simulink model "norton_5_nl_push_pull"  (Simulink 7.4)
settings: Solver=ode23t  StartTime=0.0  StopTime=1e-4  MaxStep=10e-9  RelTol=1e-4
InitFcn:
  | M=3;
  | N=M^2-M-1;
  | 
  | L1=1e-6;
  | R1=0.1;
  | L2=(M^2)*L1;
  | R2=R1*M;
  | L3=(N^2)*L1;
  | R3=R1*N;
  | 
  | K=0.999;
  | M12 = K*sqrt(L1*L2);
  | M13 = K*sqrt(L1*L3);
  | M23 = K*sqrt(L2*L3);
  | 
  | % center tapped input transformer
  | Kio = 0.999;
  | Lio1 = 4e-6;
  | Lio2   = Lio1*(0.5^2);
  | Lio3   = Lio2;
  | Mio12 = Kio*sqrt(Lio1*Lio2);
  | Mio13 = Kio*sqrt(Lio1*Lio3);
  | Mio23 = Kio*sqrt(Lio2*Lio3);
  | Rio = 1;
  | 
  | % Passive Augmentation Transformer
  | La1 = 1e-6;
  | Ka=0.9999;
  | Tratio = 5;
  | La2 = La1*(Tratio^2);
  | Ma12 = Ka*Tratio*La1;
  | Ra1=0.1;
  | Ra2=Tratio*Ra1;
StopFcn:
  | if ~SPECTRUM_FLAG
  |      %% plot measured sparameters using RFTB
  |     amp=rfdata.data;
  |     amp.Freq=spar(:,1);
  | %%
  |     amp.S_parameters=complex(zeros(2,2,length(amp.Freq)));
  |    if spar(1,6)==1
  |       amp.S_Parameters(1,1,:)=spar(:,2)+1i*spar(:,3);
  |       amp.S_Parameters(2,1,:)=spar(:,4)+1i*spar(:,5);
  |       subplot(2,1,1);
  |       hplot1= smith(amp,'s11')
  |       subplot(2,1,2);
  |       hplot2 = plot(amp,'s21');
  |       axis([amp.Freq(1)/1e6,amp.Freq(end)/1e6,0,10]);
  |    else
  |       amp.S_Parameters(2,2,:)=spar(:,2)+1i*spar(:,3);
  |       amp.S_Parameters(1,2,:)=spar(:,4)+1i*spar(:,5);
  |       subplot(2,1,1);
  |       hplot1= smith(amp,'s22')
  |       subplot(2,1,2);
  |       hplot2 = plot(amp,'s12');
  |    end;
  | end
undefined symbols (not defined in the file or in its folder): Fs, magnitude, One, sided
libraries: powerlib x65, dspindex x12, dspsigops x6, dspbuff3 x5, dsparch4 x5, simulink x4, dspxfrm3 x4, dsparch3 x4, dspsnks4 x3, dspmtrx3 x2, dspstat3 x1
(part 1 of 2)
settings Model: Creator=Dick  LastModifiedBy=Dick

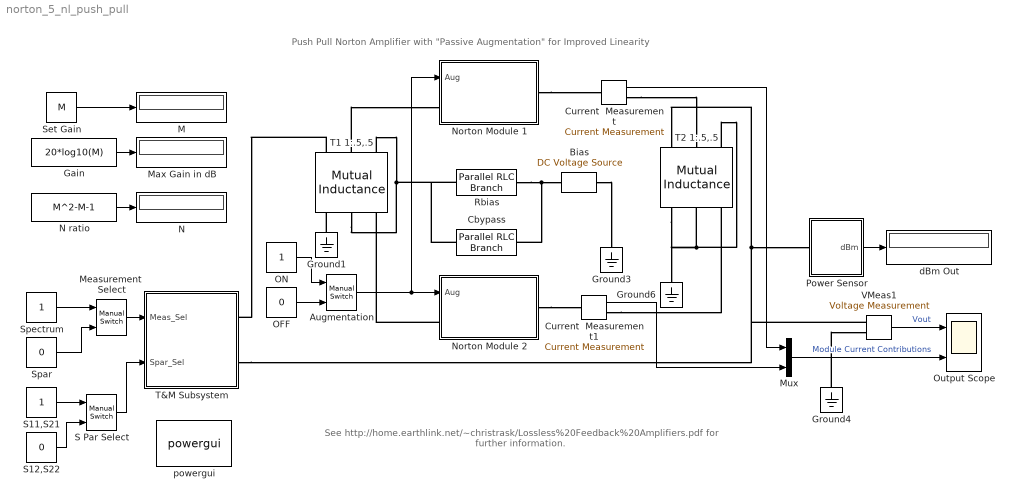
== system norton_5_nl_push_pull ==
  note: Push Pull Norton Amplifier with "Passive Augmentation" for Improved Linearity
  note: See http://home.earthlink.net/~christrask/Lossless%20Feedback%20Amplifiers.pdf
      | for further information.
  Augmentation : simulink/Signal Routing/Manual Switch  SystemSampleTime=-1  sw=0  action=0  varsize=off
  Bias : powerlib/Electrical Sources/DC Voltage Source  DialogController=POWERSYS.PowerSysDialog  SystemSampleTime=-1  Amplitude=3  Measurements=None
  Cbypass : powerlib/Elements/Parallel RLC Branch  DialogController=POWERSYS.PowerSysDialog  PhysicalDomain=powersysdomain  SubClassName=unknown  LeftPortType=p1  RightPortType=p1  LConnTagsString=a  RConnTagsString=__new0  BranchType=C  Resistance=.01  Inductance=1e-3  SetiL0=off  InitialCurrent=0  Capacitance=1e-7  Setx0=off  InitialVoltage=0  Measurements=None
  Current  Measurement : powerlib/Measurements/Current Measurement  DialogController=POWERSYS.PowerSysDialog  SystemSampleTime=-1  PhasorSimulation=off  OutputType=Complex  PSBequivalent=0
  Current  Measurement1 : powerlib/Measurements/Current Measurement  DialogController=POWERSYS.PowerSysDialog  SystemSampleTime=-1  PhasorSimulation=off  OutputType=Complex  PSBequivalent=0
  Gain : Constant  Value=20*log10(M)  OutDataType=fixdt(1, 16)  OutScaling=2^0
  Ground{1,3..4,6} (4 alike) : powerlib/Elements/Ground  DialogController=POWERSYS.PowerSysDialog  PhysicalDomain=powersysdomain  SubClassName=unknown  LeftPortType=p1  RightPortType=p1  LConnTagsString=a
  M : Display
  Max Gain in dB : Display
  Measurement  Select : simulink/Signal Routing/Manual Switch  SystemSampleTime=-1  sw=1  action=0  varsize=off
  Mux : Mux  Inputs=2
  N : Display
  N ratio : Constant  Value=M^2-M-1  OutDataType=fixdt(1, 16)  OutScaling=2^0
  Norton Module 1 : Subsystem
  Norton Module 2 : Subsystem
  OFF : Constant  Value=0  OutDataType=fixdt(1, 16)  OutScaling=2^0
  ON : Constant  OutDataType=fixdt(1, 16)  OutScaling=2^0
  Output Scope : Scope  NumInputPorts=2
      settings: TimeRange=5.999999999999993e-007  YMin=-30~-0.3  YMax=30~1.2
  Power Sensor : Subsystem
  Rbias : powerlib/Elements/Parallel RLC Branch  DialogController=POWERSYS.PowerSysDialog  PhysicalDomain=powersysdomain  SubClassName=unknown  LeftPortType=p1  RightPortType=p1  LConnTagsString=a  RConnTagsString=__new0  BranchType=R  Resistance=50/2  Inductance=1e-3  SetiL0=off  InitialCurrent=0  Capacitance=1e-6  Setx0=off  InitialVoltage=0  Measurements=None
  S Par Select : simulink/Signal Routing/Manual Switch  SystemSampleTime=-1  sw=1  action=0  varsize=off
  S11,S21 : Constant  OutDataType=fixdt(1, 16)  OutScaling=2^0
  S12,S22 : Constant  Value=0  OutDataType=fixdt(1, 16)  OutScaling=2^0
  Set Gain : Constant  Value=M  OutDataType=fixdt(1, 16)  OutScaling=2^0
  Spar : Constant  Value=0  OutDataTypeMode=boolean  OutDataType=fixdt(1, 16)  OutScaling=2^0  OutDataTypeStr=boolean
  Spectrum : Constant  OutDataTypeMode=boolean  OutDataType=fixdt(1, 16)  OutScaling=2^0  OutDataTypeStr=boolean
  T&M Subsystem : Subsystem
  T1 1:.5,.5 : powerlib/Elements/Mutual Inductance  DialogController=POWERSYS.PowerSysDialog  PhysicalDomain=powersysdomain  SubClassName=unknown  LeftPortType=p1  RightPortType=p1  LConnTagsString=a|b|c  RConnTagsString=A|B|C  TypeOfMutual=Generalized mutual inductance  NumberOfWindings=3  SelfImpedance1=[R1,L1]  SelfImpedance2=[R2,L2]  ThreeWindings=on  SelfImpedance3=[]  MutualImpedance=[1.0 1.0e-03]  InductanceMatrix=[Lio1 Mio12 Mio13; Mio12 Lio2 Mio23; Mio13 Mio23 Lio3];  ResistanceMatrix="[1  0 0 ; 0 1 0 ; 0 0 1]*Rio;"  Measurements=None
      settings: AttributesFormatString=\n
  T2 1:.5,.5 : powerlib/Elements/Mutual Inductance  DialogController=POWERSYS.PowerSysDialog  PhysicalDomain=powersysdomain  SubClassName=unknown  LeftPortType=p1  RightPortType=p1  LConnTagsString=a|b|c  RConnTagsString=A|B|C  TypeOfMutual=Generalized mutual inductance  NumberOfWindings=3  SelfImpedance1=[R1,L1]  SelfImpedance2=[R2,L2]  ThreeWindings=on  SelfImpedance3=[]  MutualImpedance=[1.0 1.0e-03]  InductanceMatrix=[Lio1 Mio12 Mio13; Mio12 Lio2 Mio23; Mio13 Mio23 Lio3];  ResistanceMatrix="[1  0 0 ; 0 1 0 ; 0 0 1]*Rio;"  Measurements=None
      settings: AttributesFormatString=\n
  VMeas1 : powerlib/Measurements/Voltage Measurement  DialogController=POWERSYS.PowerSysDialog  SystemSampleTime=-1  PhasorSimulation=off  OutputType=Complex  PSBequivalent=0
  dBm Out : Display
  powergui : powerlib/powergui  Priority=1  SystemSampleTime=-1  SimulationMode=Continuous  SampleTime=50e-6  frequency=60  SPID=off  DisableSnubberDevices=off  DisableRonSwitches=off  DisableVfSwitches=off  SwTol=0  Interpol=off  frequencyindice=0  echomessages=off  HookPort=off  DisplayEquations=off  FunctionMessages=off  EnableUseOfTLC=off  x0status=blocks  RestoreLinks=warning  Frange=[0:2:500]  Ylog=off  Xlog=on  ShowGrid=off  save=off  variable=ZData  ZoomFFT=on  StartTime=0.0  cycles=1  DisplayStyle=1  fundamental=60  FreqAxis=off  MaxFrequency=1000  frequencyindicesteady=1  RmsSteady=1  display=off  Ts=0  methode=off
  wires:
  Set Gain/1 -> M/1
  N ratio/1 -> N/1
  Gain/1 -> Max Gain in dB/1
  ON/1 -> Augmentation/1
  OFF/1 -> Augmentation/2
  Augmentation/1 -> Norton Module 1/1(Aug), Norton Module 2/1(Aug)
  Measurement  Select/1 -> T&M Subsystem/1(Meas_Sel)
  Spar/1 -> Measurement  Select/2
  Spectrum/1 -> Measurement  Select/1
  S Par Select/1 -> T&M Subsystem/2(Spar_Sel)
  S11,S21/1 -> S Par Select/1
  S12,S22/1 -> S Par Select/2
  Current  Measurement/1 -> Mux/1
  Current  Measurement1/1 -> Mux/2
  Mux/1 -> Output Scope/2  "Module Current Contributions"
  VMeas1/1 -> Output Scope/1  "Vout"
  Power Sensor/1(dBm) -> dBm Out/1
  connections:
  Ground1/LConn1 -- T1 1:.5,.5/RConn1
  T1 1:.5,.5/LConn2 -- Norton Module 1/LConn1
  Bias/LConn1 -- Ground3/LConn1
  Norton Module 2/LConn1 -- T1 1:.5,.5/RConn3
  T1 1:.5,.5/LConn3 -- T1 1:.5,.5/RConn2 -- Rbias/LConn1 -- Cbypass/RConn1
  Rbias/RConn1 -- Bias/RConn1 -- Cbypass/LConn1
  T2 1:.5,.5/RConn1 -- Ground6/LConn1 -- T2 1:.5,.5/RConn2 -- T2 1:.5,.5/LConn3
  T1 1:.5,.5/LConn1 -- T&M Subsystem/RConn1
  T&M Subsystem/RConn2 -- VMeas1/LConn1 -- T2 1:.5,.5/LConn1 -- Power Sensor/LConn1
  Norton Module 1/RConn1 -- Current  Measurement/LConn1
  Current  Measurement/RConn1 -- T2 1:.5,.5/LConn2
  Norton Module 2/RConn1 -- Current  Measurement1/LConn1
  Current  Measurement1/RConn1 -- T2 1:.5,.5/RConn3
  Ground4/LConn1 -- VMeas1/LConn2

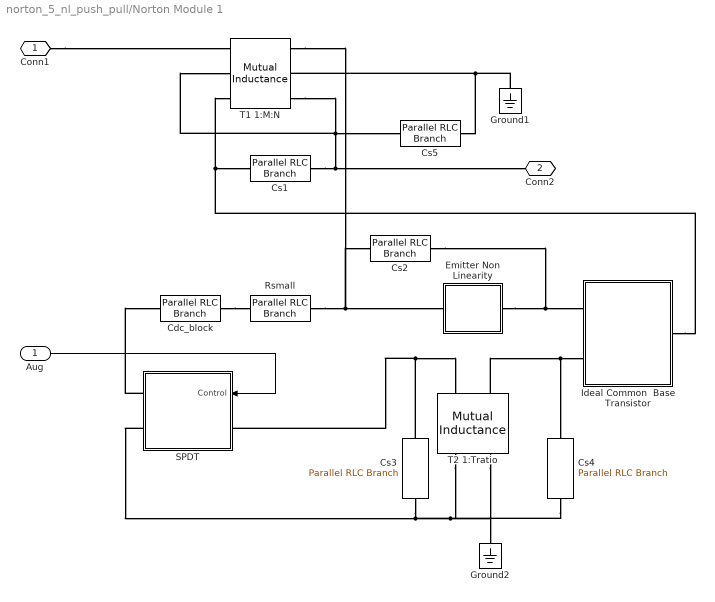
== system norton_5_nl_push_pull/Norton Module 1 ==
  Aug : Inport  OutDataType=fixdt(1, 16)  OutScaling=2^0
  Cdc_block : powerlib/Elements/Parallel RLC Branch  DialogController=POWERSYS.PowerSysDialog  PhysicalDomain=powersysdomain  SubClassName=unknown  LeftPortType=p1  RightPortType=p1  LConnTagsString=a  RConnTagsString=__new0  BranchType=C  Resistance=5000  Inductance=1e-3  SetiL0=off  InitialCurrent=0  Capacitance=1e-8  Setx0=off  InitialVoltage=0  Measurements=None
  Cs1 : powerlib/Elements/Parallel RLC Branch  DialogController=POWERSYS.PowerSysDialog  PhysicalDomain=powersysdomain  SubClassName=unknown  LeftPortType=p1  RightPortType=p1  LConnTagsString=a  RConnTagsString=__new0  BranchType=C  Resistance=5000  Inductance=1e-3  SetiL0=off  InitialCurrent=0  Capacitance=1e-12  Setx0=off  InitialVoltage=0  Measurements=None
  Cs2 : powerlib/Elements/Parallel RLC Branch  DialogController=POWERSYS.PowerSysDialog  PhysicalDomain=powersysdomain  SubClassName=unknown  LeftPortType=p1  RightPortType=p1  LConnTagsString=a  RConnTagsString=__new0  BranchType=C  Resistance=5000  Inductance=1e-3  SetiL0=off  InitialCurrent=0  Capacitance=1e-12  Setx0=off  InitialVoltage=0  Measurements=None
  Cs3 : powerlib/Elements/Parallel RLC Branch  DialogController=POWERSYS.PowerSysDialog  PhysicalDomain=powersysdomain  SubClassName=unknown  LeftPortType=p1  RightPortType=p1  LConnTagsString=a  RConnTagsString=__new0  BranchType=C  Resistance=.01  Inductance=1e-3  SetiL0=off  InitialCurrent=0  Capacitance=1e-12  Setx0=off  InitialVoltage=0  Measurements=None
  Cs4 : powerlib/Elements/Parallel RLC Branch  DialogController=POWERSYS.PowerSysDialog  PhysicalDomain=powersysdomain  SubClassName=unknown  LeftPortType=p1  RightPortType=p1  LConnTagsString=a  RConnTagsString=__new0  BranchType=C  Resistance=.01  Inductance=1e-3  SetiL0=off  InitialCurrent=0  Capacitance=1e-12  Setx0=off  InitialVoltage=0  Measurements=None
  Cs5 : powerlib/Elements/Parallel RLC Branch  DialogController=POWERSYS.PowerSysDialog  PhysicalDomain=powersysdomain  SubClassName=unknown  LeftPortType=p1  RightPortType=p1  LConnTagsString=a  RConnTagsString=__new0  BranchType=C  Resistance=5000  Inductance=1e-3  SetiL0=off  InitialCurrent=0  Capacitance=1e-12  Setx0=off  InitialVoltage=0  Measurements=None
  Emitter Non Linearity : Subsystem  mask{Is=1e-7}
      mask prompts: Is "Saturation Current"
      mask Display: plot(-140,-140,150,140,2*[30,30,59,30,30,0]-75,(2*[71,50,72,92,71,71]-92),2*[59,59]-75,(2*[50,93]-92),[116,59]-16,(2*[71,71]-90));
  Ground1 : powerlib/Elements/Ground  DialogController=POWERSYS.PowerSysDialog  PhysicalDomain=powersysdomain  SubClassName=unknown  LeftPortType=p1  RightPortType=p1  LConnTagsString=a
  Ground2 : powerlib/Elements/Ground  DialogController=POWERSYS.PowerSysDialog  PhysicalDomain=powersysdomain  SubClassName=unknown  LeftPortType=p1  RightPortType=p1  LConnTagsString=a
  Ideal Common  Base Transistor : Subsystem
  Rsmall : powerlib/Elements/Parallel RLC Branch  DialogController=POWERSYS.PowerSysDialog  PhysicalDomain=powersysdomain  SubClassName=unknown  LeftPortType=p1  RightPortType=p1  LConnTagsString=a  RConnTagsString=__new0  BranchType=R  Resistance=3.3  Inductance=1e-3  SetiL0=off  InitialCurrent=0  Capacitance=1e-12  Setx0=off  InitialVoltage=0  Measurements=None
  SPDT : Subsystem
  T1 1:M:N : powerlib/Elements/Mutual Inductance  DialogController=POWERSYS.PowerSysDialog  PhysicalDomain=powersysdomain  SubClassName=unknown  LeftPortType=p1  RightPortType=p1  LConnTagsString=a|b|c  RConnTagsString=A|B|C  TypeOfMutual=Generalized mutual inductance  NumberOfWindings=3  SelfImpedance1=[R1,L1]  SelfImpedance2=[R2,L2]  ThreeWindings=on  SelfImpedance3=[]  MutualImpedance=[1.0 1.0e-03]  InductanceMatrix="[L1 M12 M13;  M12 L2 M23; M13 M23 L3];"  ResistanceMatrix=[R1 0 0; 0 R2 0; 0 0 R3 ];  Measurements=None
      settings: AttributesFormatString=\n
  T2 1:Tratio : powerlib/Elements/Mutual Inductance  DialogController=POWERSYS.PowerSysDialog  PhysicalDomain=powersysdomain  SubClassName=unknown  LeftPortType=p1  RightPortType=p1  LConnTagsString=a|b  RConnTagsString=A|B  TypeOfMutual=Generalized mutual inductance  NumberOfWindings=2  SelfImpedance1=[R1,L1]  SelfImpedance2=[R2,L2]  ThreeWindings=on  SelfImpedance3=[]  MutualImpedance=[1.0 1.0e-03]  InductanceMatrix=[La1 -Ma12;-Ma12 La2];  ResistanceMatrix=[Ra1 0 ; 0 Ra2 ];  Measurements=None
      settings: AttributesFormatString=\n
  Conn1 : PMIOPort  Port=1  Side=Left
  Conn2 : PMIOPort  Port=2  Side=Right
  wires:
  Aug/1 -> SPDT/1(Control)
  connections:
  SPDT/RConn1 -- Cdc_block/LConn1
  Cdc_block/RConn1 -- Rsmall/RConn1
  Ideal Common  Base Transistor/RConn1 -- Cs1/LConn1 -- T1 1:M:N/LConn3
  T1 1:M:N/RConn3 -- Cs1/RConn1 -- Conn2/RConn1 -- T1 1:M:N/LConn2 -- Cs5/LConn1
  Rsmall/LConn1 -- Emitter Non Linearity/LConn1 -- Cs2/LConn1 -- T1 1:M:N/RConn1
  Emitter Non Linearity/RConn1 -- Cs2/RConn1 -- Ideal Common  Base Transistor/LConn1
  Cs3/LConn1 -- T2 1:Tratio/LConn1 -- SPDT/LConn1
  Cs3/RConn1 -- Ground2/LConn1 -- T2 1:Tratio/RConn2 -- Cs4/RConn1 -- T2 1:Tratio/RConn1 -- SPDT/RConn2
  T2 1:Tratio/LConn2 -- Cs4/LConn1 -- Ideal Common  Base Transistor/LConn2
  Ground1/LConn1 -- T1 1:M:N/RConn2 -- Cs5/RConn1
  Conn1/RConn1 -- T1 1:M:N/LConn1

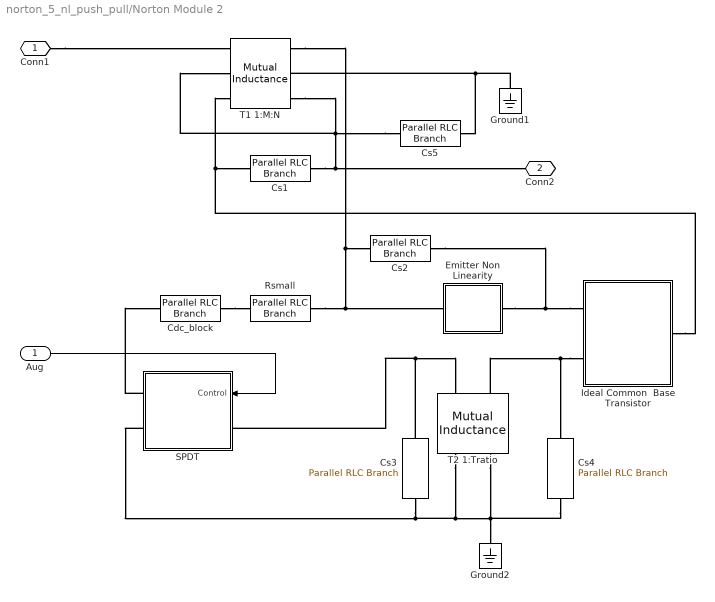
== system norton_5_nl_push_pull/Norton Module 2 ==
  Aug : Inport  OutDataType=fixdt(1, 16)  OutScaling=2^0
  Cdc_block : powerlib/Elements/Parallel RLC Branch  DialogController=POWERSYS.PowerSysDialog  PhysicalDomain=powersysdomain  SubClassName=unknown  LeftPortType=p1  RightPortType=p1  LConnTagsString=a  RConnTagsString=__new0  BranchType=C  Resistance=5000  Inductance=1e-3  SetiL0=off  InitialCurrent=0  Capacitance=1e-8  Setx0=off  InitialVoltage=0  Measurements=None
  Cs1 : powerlib/Elements/Parallel RLC Branch  DialogController=POWERSYS.PowerSysDialog  PhysicalDomain=powersysdomain  SubClassName=unknown  LeftPortType=p1  RightPortType=p1  LConnTagsString=a  RConnTagsString=__new0  BranchType=C  Resistance=5000  Inductance=1e-3  SetiL0=off  InitialCurrent=0  Capacitance=1e-12  Setx0=off  InitialVoltage=0  Measurements=None
  Cs2 : powerlib/Elements/Parallel RLC Branch  DialogController=POWERSYS.PowerSysDialog  PhysicalDomain=powersysdomain  SubClassName=unknown  LeftPortType=p1  RightPortType=p1  LConnTagsString=a  RConnTagsString=__new0  BranchType=C  Resistance=5000  Inductance=1e-3  SetiL0=off  InitialCurrent=0  Capacitance=1e-12  Setx0=off  InitialVoltage=0  Measurements=None
  Cs3 : powerlib/Elements/Parallel RLC Branch  DialogController=POWERSYS.PowerSysDialog  PhysicalDomain=powersysdomain  SubClassName=unknown  LeftPortType=p1  RightPortType=p1  LConnTagsString=a  RConnTagsString=__new0  BranchType=C  Resistance=.01  Inductance=1e-3  SetiL0=off  InitialCurrent=0  Capacitance=1e-12  Setx0=off  InitialVoltage=0  Measurements=None
  Cs4 : powerlib/Elements/Parallel RLC Branch  DialogController=POWERSYS.PowerSysDialog  PhysicalDomain=powersysdomain  SubClassName=unknown  LeftPortType=p1  RightPortType=p1  LConnTagsString=a  RConnTagsString=__new0  BranchType=C  Resistance=.01  Inductance=1e-3  SetiL0=off  InitialCurrent=0  Capacitance=1e-12  Setx0=off  InitialVoltage=0  Measurements=None
  Cs5 : powerlib/Elements/Parallel RLC Branch  DialogController=POWERSYS.PowerSysDialog  PhysicalDomain=powersysdomain  SubClassName=unknown  LeftPortType=p1  RightPortType=p1  LConnTagsString=a  RConnTagsString=__new0  BranchType=C  Resistance=5000  Inductance=1e-3  SetiL0=off  InitialCurrent=0  Capacitance=1e-12  Setx0=off  InitialVoltage=0  Measurements=None
  Emitter Non Linearity : Subsystem  mask{Is=1e-7}
      mask prompts: Is "Saturation Current"
      mask Display: plot(-140,-140,150,140,2*[30,30,59,30,30,0]-75,(2*[71,50,72,92,71,71]-92),2*[59,59]-75,(2*[50,93]-92),[116,59]-16,(2*[71,71]-90));
  Ground1 : powerlib/Elements/Ground  DialogController=POWERSYS.PowerSysDialog  PhysicalDomain=powersysdomain  SubClassName=unknown  LeftPortType=p1  RightPortType=p1  LConnTagsString=a
  Ground2 : powerlib/Elements/Ground  DialogController=POWERSYS.PowerSysDialog  PhysicalDomain=powersysdomain  SubClassName=unknown  LeftPortType=p1  RightPortType=p1  LConnTagsString=a
  Ideal Common  Base Transistor : Subsystem
  Rsmall : powerlib/Elements/Parallel RLC Branch  DialogController=POWERSYS.PowerSysDialog  PhysicalDomain=powersysdomain  SubClassName=unknown  LeftPortType=p1  RightPortType=p1  LConnTagsString=a  RConnTagsString=__new0  BranchType=R  Resistance=3.3  Inductance=1e-3  SetiL0=off  InitialCurrent=0  Capacitance=1e-12  Setx0=off  InitialVoltage=0  Measurements=None
  SPDT : Subsystem
  T1 1:M:N : powerlib/Elements/Mutual Inductance  DialogController=POWERSYS.PowerSysDialog  PhysicalDomain=powersysdomain  SubClassName=unknown  LeftPortType=p1  RightPortType=p1  LConnTagsString=a|b|c  RConnTagsString=A|B|C  TypeOfMutual=Generalized mutual inductance  NumberOfWindings=3  SelfImpedance1=[R1,L1]  SelfImpedance2=[R2,L2]  ThreeWindings=on  SelfImpedance3=[]  MutualImpedance=[1.0 1.0e-03]  InductanceMatrix="[L1 M12 M13;  M12 L2 M23; M13 M23 L3];"  ResistanceMatrix=[R1 0 0; 0 R2 0; 0 0 R3 ];  Measurements=None
      settings: AttributesFormatString=\n
  T2 1:Tratio : powerlib/Elements/Mutual Inductance  DialogController=POWERSYS.PowerSysDialog  PhysicalDomain=powersysdomain  SubClassName=unknown  LeftPortType=p1  RightPortType=p1  LConnTagsString=a|b  RConnTagsString=A|B  TypeOfMutual=Generalized mutual inductance  NumberOfWindings=2  SelfImpedance1=[R1,L1]  SelfImpedance2=[R2,L2]  ThreeWindings=on  SelfImpedance3=[]  MutualImpedance=[1.0 1.0e-03]  InductanceMatrix=[La1 -Ma12;-Ma12 La2];  ResistanceMatrix=[Ra1 0 ; 0 Ra2 ];  Measurements=None
      settings: AttributesFormatString=\n
  Conn1 : PMIOPort  Port=1  Side=Left
  Conn2 : PMIOPort  Port=2  Side=Right
  wires:
  Aug/1 -> SPDT/1(Control)
  connections:
  Conn1/RConn1 -- T1 1:M:N/LConn1
  Cs5/RConn1 -- T1 1:M:N/RConn2 -- Ground1/LConn1
  Ideal Common  Base Transistor/LConn2 -- Cs4/LConn1 -- T2 1:Tratio/LConn2
  SPDT/RConn2 -- T2 1:Tratio/RConn1 -- Cs4/RConn1 -- T2 1:Tratio/RConn2 -- Ground2/LConn1 -- Cs3/RConn1
  SPDT/LConn1 -- T2 1:Tratio/LConn1 -- Cs3/LConn1
  Ideal Common  Base Transistor/LConn1 -- Cs2/RConn1 -- Emitter Non Linearity/RConn1
  T1 1:M:N/RConn1 -- Cs2/LConn1 -- Emitter Non Linearity/LConn1 -- Rsmall/LConn1
  Cs5/LConn1 -- T1 1:M:N/LConn2 -- Conn2/RConn1 -- Cs1/RConn1 -- T1 1:M:N/RConn3
  T1 1:M:N/LConn3 -- Cs1/LConn1 -- Ideal Common  Base Transistor/RConn1
  Cdc_block/RConn1 -- Rsmall/RConn1
  SPDT/RConn1 -- Cdc_block/LConn1

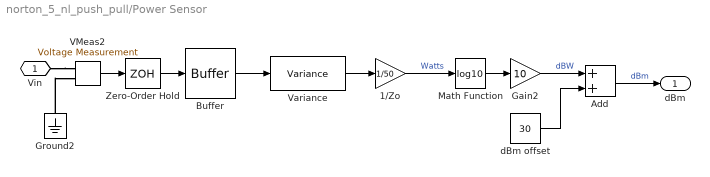
== system norton_5_nl_push_pull/Power Sensor ==
  1/Zo : Gain  Gain=1/50  ParameterDataType=fixdt(1, 16)  ParameterScaling=2^0  OutDataType=fixdt(1, 16)  OutScaling=2^0
  Add : Sum  OutDataType=fixdt(1, 16)  OutScaling=2^-10
  Buffer : dspbuff3/Buffer  N=1000  V=0  ic=0
  Gain2 : Gain  Gain=10  ParameterDataType=fixdt(1, 16)  ParameterScaling=2^0  OutDataType=fixdt(1, 16)  OutScaling=2^0
  Ground2 : powerlib/Elements/Ground  DialogController=POWERSYS.PowerSysDialog  PhysicalDomain=powersysdomain  SubClassName=unknown  LeftPortType=p1  RightPortType=p1  LConnTagsString=a
  Math Function : Math  Operator=log10  OutDataType=fixdt(1, 16)  OutScaling=2^0  SaturateOnIntegerOverflow=on
  VMeas2 : powerlib/Measurements/Voltage Measurement  DialogController=POWERSYS.PowerSysDialog  SystemSampleTime=-1  PhasorSimulation=off  OutputType=Complex  PSBequivalent=0
  Variance : dspstat3/Variance  DialogController=dspDDGCreate  DialogControllerArgs=DataTag0  run=off  reset_popup=None  directionMode=Each column  dimension=1  treatSBRowAsCol=on  roiEnable=off  roiType=Rectangles  roiPortion=Entire ROI  roiOutput=Individual statistics for each ROI  roiFlag=off  roundingMode=Floor  overflowMode=off
  Zero-Order Hold : ZeroOrderHold  SampleTime=1/200e6
  dBm offset : Constant  Value=30  OutDataTypeMode=double  OutDataType=fixdt(1, 16)  OutScaling=2^0  OutDataTypeStr=double
  Vin : PMIOPort  Port=1  Side=Left
  dBm : Outport
  wires:
  Zero-Order Hold/1 -> Buffer/1
  Buffer/1 -> Variance/1
  Variance/1 -> 1/Zo/1
  1/Zo/1 -> Math Function/1  "Watts"
  VMeas2/1 -> Zero-Order Hold/1
  Math Function/1 -> Gain2/1
  Gain2/1 -> Add/1  "dBW"
  dBm offset/1 -> Add/2
  Add/1 -> dBm/1  "dBm"
  connections:
  Ground2/LConn1 -- VMeas2/LConn2
  Vin/RConn1 -- VMeas2/LConn1

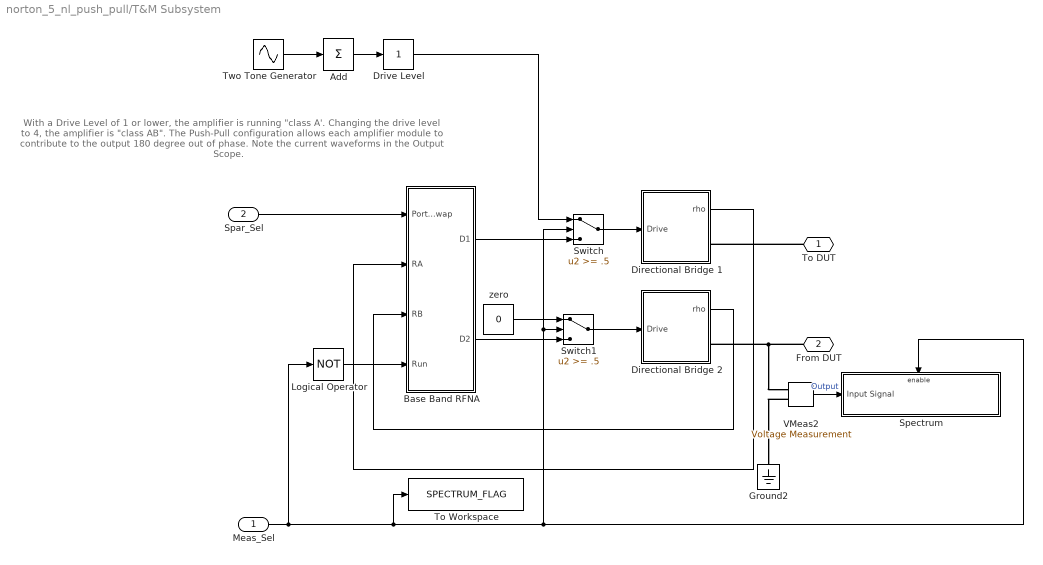
== system norton_5_nl_push_pull/T&M Subsystem ==
  note: With a Drive Level of 1 or lower, the amplifier is running "class A'.
      |
      | Changing the drive level to 4, the amplifier is "class AB".
      | The Push-Pull configuration allows each amplifier module
      | to contribute to the output 180 degree out of phase.
      | Note the current waveforms in the Output Scope.
  Meas_Sel : Inport  OutDataType=fixdt(1, 16)  OutScaling=2^0
  Spar_Sel : Inport  Port=2  OutDataType=fixdt(1, 16)  OutScaling=2^0
  Add : Sum  Inputs=+  OutDataType=fixdt(1, 16)  OutScaling=2^-10
  Base Band RFNA : Subsystem  Description=Spectrum Analyzer  mask{BW=100e6, Frame_Size=256}
      mask prompts: BW "Bandwidth"; Frame_Size "FFT SIze (256,512,1024 etc)"
  Directional Bridge 1 : Subsystem  mask{Zo=50}
      mask prompts: Zo "Zo="
  Directional Bridge 2 : Subsystem  mask{Zo=50}
      mask prompts: Zo "Zo="
  Drive Level : simulink/Math Operations/Slider Gain  SystemSampleTime=-1  low=0.5  gain=1  high=4
  Ground2 : powerlib/Elements/Ground  DialogController=POWERSYS.PowerSysDialog  PhysicalDomain=powersysdomain  SubClassName=unknown  LeftPortType=p1  RightPortType=p1  LConnTagsString=a
  Logical Operator : Logic  Operator=NOT  AllPortsSameDT=off  OutDataTypeMode=boolean  LogicDataType=fixdt(0, 8)  OutDataTypeStr=boolean
  Spectrum : Subsystem  Description=Spectrum Analyzer  mask{BW=100e6, Zo=50}
      mask prompts: BW "Bandwidth"; Zo "Load Zo"
      mask Display: fprintf('Baseband Spectrum Analyzer \n  BW=%7.2f MHz', BW/1e6)
  Switch : Switch  Threshold=.5  OutDataType=fixdt(1, 16)  OutScaling=2^0
  Switch1 : Switch  Threshold=.5  OutDataType=fixdt(1, 16)  OutScaling=2^0
  To Workspace : ToWorkspace  VariableName=SPECTRUM_FLAG  SampleTime=-1  SaveFormat=Array
      settings: MaxDataPoints=1
  Two Tone Generator : Sin  Amplitude=2*sqrt(2)  Bias=0  Frequency=[20e6 25e6]*2*pi  Phase=0  Samples=10  SampleTime=0  Offset=0
  VMeas2 : powerlib/Measurements/Voltage Measurement  DialogController=POWERSYS.PowerSysDialog  SystemSampleTime=-1  PhasorSimulation=off  OutputType=Complex  PSBequivalent=0
  zero : Constant  Value=0  OutDataTypeMode=boolean  OutDataType=fixdt(1, 16)  OutScaling=2^0  OutDataTypeStr=boolean
  To DUT : PMIOPort  Port=1  Side=Right
  From DUT : PMIOPort  Port=2  Side=Right
  wires:
  Two Tone Generator/1 -> Add/1
  Directional Bridge 1/1(rho) -> Base Band RFNA/2(RA)
  Directional Bridge 2/1(rho) -> Base Band RFNA/3(RB)
  VMeas2/1 -> Spectrum/1(Input Signal)  "Output"
  Base Band RFNA/1(D1) -> Switch/3
  Switch/1 -> Directional Bridge 1/1(Drive)
  Add/1 -> Drive Level/1
  Switch1/1 -> Directional Bridge 2/1(Drive)
  Base Band RFNA/2(D2) -> Switch1/3
  zero/1 -> Switch1/1
  Logical Operator/1 -> Base Band RFNA/4(Run)
  Meas_Sel/1 -> Logical Operator/1, Switch1/2, Switch/2, Spectrum/Enable, To Workspace/1
  Spar_Sel/1 -> Base Band RFNA/1(Port Swap)
  Drive Level/1 -> Switch/1
  connections:
  From DUT/RConn1 -- Directional Bridge 2/RConn1 -- VMeas2/LConn1
  VMeas2/LConn2 -- Ground2/LConn1
  To DUT/RConn1 -- Directional Bridge 1/RConn1

== system norton_5_nl_push_pull/Norton Module 1/Emitter Non Linearity ==
  Diode Equation : Fcn  Expr="Is* (exp(u /.025)  -1  );  % ideal diode equation @ room temp"
  "Vf " : powerlib/Measurements/Voltage Measurement  Tag=PoWeRsYsTeMmEaSuReMeNt  DialogController=POWERSYS.PowerSysDialog  SystemSampleTime=-1  PhasorSimulation=off  OutputType=Magnitude  PSBequivalent=0
  ik1 : powerlib/Electrical Sources/Controlled Current Source  Description=source block  DialogController=POWERSYS.PowerSysDialog  SystemSampleTime=-1  Initialize=on  Source_Type=AC  Amplitude=0  Phase=0  Frequency=0  Measurements=None
      settings: AttributesFormatString=\n
  Anode : PMIOPort  Tag=PMCPort  Port=1  Side=Left
  "cathode " : PMIOPort  Tag=PMCPort  Port=2  Side=Right
  wires:
  "Vf "/1 -> Diode Equation/1
  Diode Equation/1 -> ik1/1
  connections:
  "Vf "/LConn1 -- Anode/RConn1 -- ik1/LConn1
  ik1/RConn1 -- "cathode "/RConn1 -- "Vf "/LConn2

== system norton_5_nl_push_pull/Norton Module 1/Ideal Common  Base Transistor ==
  Alpha : Gain  Gain=.99  ParameterDataType=fixdt(1, 16)  ParameterScaling=2^0  OutDataType=fixdt(1, 16)  OutScaling=2^0
  Controlled Current Source : powerlib/Electrical Sources/Controlled Current Source  DialogController=POWERSYS.PowerSysDialog  SystemSampleTime=-1  Initialize=off  Source_Type=DC  Amplitude=0  Phase=0  Frequency=0  Measurements=None
  Current  Measurement : powerlib/Measurements/Current Measurement  DialogController=POWERSYS.PowerSysDialog  SystemSampleTime=-1  PhasorSimulation=off  OutputType=Complex  PSBequivalent=0
  Emitter : PMIOPort  Port=1  Side=Left
  Collector : PMIOPort  Port=2  Side=Right
  Base : PMIOPort  Port=3  Side=Left
  wires:
  Current  Measurement/1 -> Alpha/1
  Alpha/1 -> Controlled Current Source/1
  connections:
  Base/RConn1 -- Current  Measurement/RConn1 -- Controlled Current Source/LConn1
  Collector/RConn1 -- Controlled Current Source/RConn1
  Emitter/RConn1 -- Current  Measurement/LConn1

== system norton_5_nl_push_pull/Norton Module 1/SPDT ==
  Control : Inport
  Ideal Switch : powerlib/Power Electronics/Ideal Switch  DialogController=POWERSYS.PowerSysDialog  SystemSampleTime=-1  Ron=10  Lon=0  IC=0  Rs=inf  Cs=0  Measurements=off
  Ideal Switch1 : powerlib/Power Electronics/Ideal Switch  DialogController=POWERSYS.PowerSysDialog  SystemSampleTime=-1  Ron=10  Lon=0  IC=0  Rs=inf  Cs=0  Measurements=off
  Logical Operator : Logic  Operator=NOT  AllPortsSameDT=off  OutDataTypeMode=boolean  LogicDataType=fixdt(0, 8)  OutDataTypeStr=boolean
  Common : PMIOPort  Port=1  Side=Left
  NO : PMIOPort  Port=2  Side=Right
  NC : PMIOPort  Port=3  Side=Right
  wires:
  Logical Operator/1 -> Ideal Switch1/1
  Control/1 -> Logical Operator/1, Ideal Switch/1
  connections:
  Ideal Switch/LConn1 -- Common/RConn1 -- Ideal Switch1/LConn1
  NC/RConn1 -- Ideal Switch1/RConn1
  NO/RConn1 -- Ideal Switch/RConn1

== system norton_5_nl_push_pull/Norton Module 2/Emitter Non Linearity ==
  Diode Equation : Fcn  Expr="Is* (exp(u /.025)  -1  );  % ideal diode equation @ room temp"
  "Vf " : powerlib/Measurements/Voltage Measurement  Tag=PoWeRsYsTeMmEaSuReMeNt  DialogController=POWERSYS.PowerSysDialog  SystemSampleTime=-1  PhasorSimulation=off  OutputType=Magnitude  PSBequivalent=0
  ik1 : powerlib/Electrical Sources/Controlled Current Source  Description=source block  DialogController=POWERSYS.PowerSysDialog  SystemSampleTime=-1  Initialize=on  Source_Type=AC  Amplitude=0  Phase=0  Frequency=0  Measurements=None
      settings: AttributesFormatString=\n
  Anode : PMIOPort  Tag=PMCPort  Port=1  Side=Left
  "cathode " : PMIOPort  Tag=PMCPort  Port=2  Side=Right
  wires:
  Diode Equation/1 -> ik1/1
  "Vf "/1 -> Diode Equation/1
  connections:
  "Vf "/LConn2 -- "cathode "/RConn1 -- ik1/RConn1
  ik1/LConn1 -- Anode/RConn1 -- "Vf "/LConn1

== system norton_5_nl_push_pull/Norton Module 2/Ideal Common  Base Transistor ==
  Alpha : Gain  Gain=.99  ParameterDataType=fixdt(1, 16)  ParameterScaling=2^0  OutDataType=fixdt(1, 16)  OutScaling=2^0
  Controlled Current Source : powerlib/Electrical Sources/Controlled Current Source  DialogController=POWERSYS.PowerSysDialog  SystemSampleTime=-1  Initialize=off  Source_Type=DC  Amplitude=0  Phase=0  Frequency=0  Measurements=None
  Current  Measurement : powerlib/Measurements/Current Measurement  DialogController=POWERSYS.PowerSysDialog  SystemSampleTime=-1  PhasorSimulation=off  OutputType=Complex  PSBequivalent=0
  Emitter : PMIOPort  Port=1  Side=Left
  Collector : PMIOPort  Port=2  Side=Right
  Base : PMIOPort  Port=3  Side=Left
  wires:
  Alpha/1 -> Controlled Current Source/1
  Current  Measurement/1 -> Alpha/1
  connections:
  Emitter/RConn1 -- Current  Measurement/LConn1
  Collector/RConn1 -- Controlled Current Source/RConn1
  Controlled Current Source/LConn1 -- Current  Measurement/RConn1 -- Base/RConn1

== system norton_5_nl_push_pull/Norton Module 2/SPDT ==
  Control : Inport
  Ideal Switch : powerlib/Power Electronics/Ideal Switch  DialogController=POWERSYS.PowerSysDialog  SystemSampleTime=-1  Ron=10  Lon=0  IC=0  Rs=inf  Cs=0  Measurements=off
  Ideal Switch1 : powerlib/Power Electronics/Ideal Switch  DialogController=POWERSYS.PowerSysDialog  SystemSampleTime=-1  Ron=10  Lon=0  IC=0  Rs=inf  Cs=0  Measurements=off
  Logical Operator : Logic  Operator=NOT  AllPortsSameDT=off  OutDataTypeMode=boolean  LogicDataType=fixdt(0, 8)  OutDataTypeStr=boolean
  Common : PMIOPort  Port=1  Side=Left
  NO : PMIOPort  Port=2  Side=Right
  NC : PMIOPort  Port=3  Side=Right
  wires:
  Control/1 -> Ideal Switch/1, Logical Operator/1
  Logical Operator/1 -> Ideal Switch1/1
  connections:
  NO/RConn1 -- Ideal Switch/RConn1
  NC/RConn1 -- Ideal Switch1/RConn1
  Ideal Switch1/LConn1 -- Common/RConn1 -- Ideal Switch/LConn1

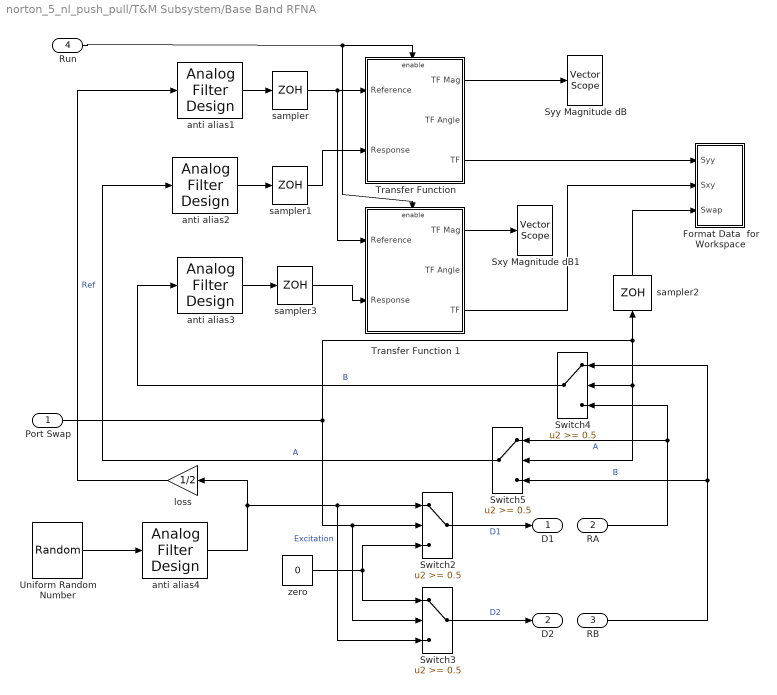
== system norton_5_nl_push_pull/T&M Subsystem/Base Band RFNA ==
  Port Swap : Inport  OutDataType=sfix(16)  OutScaling=2^0
  RA : Inport  Port=2  OutDataType=fixdt(1, 16)  OutScaling=2^0
  RB : Inport  Port=3  OutDataType=fixdt(1, 16)  OutScaling=2^0
  Run : Inport  Port=4  OutDataType=sfix(16)  OutScaling=2^0
  Format Data  for Workspace : Subsystem
  Switch{2..5} (4 alike) : Switch  Threshold=0.5  SaturateOnIntegerOverflow=on
  Sxy Magnitude dB1 : dspsnks4/Vector Scope  DialogController=dspdialog.VectorScope  DialogControllerArgs=DataTag1  ScopeProperties=on  Domain=Frequency  HorizSpan=1  DisplayProperties=off  AxisGrid=on  Memory=off  FrameNumber=on  AxisLegend=off  AxisZoom=off  OpenScopeAtSimStart=on  OpenScopeImmediately=off  FigPos=[427 57 372 236]  AxisProperties=off  XUnits=Hertz  XRange=[0...Fs/2]  InheritXIncr=on  XIncr=2*Fs  XLabel=Time  XLimit=Auto  XMin=0  XMax=1  XStart=0  YUnits=dB  YLabel=dB  LineProperties=off  LineColors=[1 0 0]|[1 0 0]  XAxisParamsVer=6.9
      settings: YMin=0  YMax=12
  Syy Magnitude dB : dspsnks4/Vector Scope  DialogController=dspdialog.VectorScope  DialogControllerArgs=DataTag2  ScopeProperties=on  Domain=Frequency  HorizSpan=1  DisplayProperties=off  AxisGrid=on  Memory=off  FrameNumber=on  AxisLegend=off  AxisZoom=off  OpenScopeAtSimStart=on  OpenScopeImmediately=off  FigPos=[45 57 372 236]  AxisProperties=off  XUnits=Hertz  XRange=[0...Fs/2]  InheritXIncr=on  XIncr=2*Fs  XLabel=Time  XLimit=Auto  XMin=0  XMax=128000000  XStart=0  YUnits=dB  YLabel=dB  LineProperties=off  LineColors=[1 0 0]|[1 0 0]  XAxisParamsVer=6.9
      settings: YMin=-40  YMax=0
  "Transfer Function " : Subsystem  mask{NFFT=Frame_Size, Navg=100, pcnt=100, unwrap_flag=on}
      mask prompts: NFFT "FFT length (power of 2):"; Navg "Spectral Averaging Factor (>=1):"; pcnt "Percentage of  Alias Free Data  (<=100)"; unwrap_flag "Unwrap Phase"
      mask Display: disp('Transfer Function \n Estimation (v2.0) ')
  Transfer Function 1 : Subsystem  mask{NFFT=Frame_Size, Navg=100, pcnt=100, unwrap_flag=on}
      mask prompts: NFFT "FFT length (power of 2):"; Navg "Spectral Averaging Factor (>=1):"; pcnt "Percentage of  Alias Free Data  (<=100)"; unwrap_flag "Unwrap Phase"
      mask Display: disp('Transfer Function \n Estimation (v2.0) ')
  Uniform Random Number : UniformRandomNumber  SampleTime=1/(2.56*BW)
  anti alias{1..4} (4 alike) : dsparch4/Analog Filter Design  method=Elliptic  filttype=Lowpass  N=8  Wlo=BW*2*pi  Whi=80  Rp=2  Rs=100
  loss : Gain  Gain=1/2  ParameterDataType=sfix(16)  ParameterScaling=2^0  OutDataType=sfix(16)  OutScaling=2^0  SaturateOnIntegerOverflow=on  OutDataTypeStr=Inherit: Same as input  ParamDataTypeStr=Inherit: Same as input
  sampler : ZeroOrderHold  SampleTime=1/(2.56*BW)
  sampler1 : ZeroOrderHold  SampleTime=1/(2.56*BW)
  sampler2 : ZeroOrderHold  SampleTime=256/(2.56*BW)
  sampler3 : ZeroOrderHold  SampleTime=1/(2.56*BW)
  zero : Constant  Value=0  OutDataType=sfix(16)  OutScaling=2^0
  D1 : Outport  OutDataType=fixdt(1, 16)  OutScaling=2^0
  D2 : Outport  Port=2  OutDataType=fixdt(1, 16)  OutScaling=2^0
  wires:
  sampler/1 -> "Transfer Function "/1(Reference), Transfer Function 1/1(Reference)
  anti alias1/1 -> sampler/1
  anti alias2/1 -> sampler1/1
  Uniform Random Number/1 -> anti alias4/1
  anti alias3/1 -> sampler3/1
  sampler3/1 -> Transfer Function 1/2(Response)
  anti alias4/1 -> loss/1, Switch3/3, Switch2/1  "Excitation"
  loss/1 -> anti alias1/1  "Ref"
  Port Swap/1 -> Switch3/2, Switch2/2, Switch4/2, Switch5/2, sampler2/1
  zero/1 -> Switch2/3, Switch3/1
  Switch2/1 -> D1/1  "D1"
  Switch3/1 -> D2/1  "D2"
  Switch5/1 -> anti alias2/1  "A"
  Switch4/1 -> anti alias3/1  "B"
  RB/1 -> Switch5/3, Switch4/1  "B"
  sampler1/1 -> "Transfer Function "/2(Response)
  "Transfer Function "/1(TF Mag) -> Syy Magnitude dB/1
  Transfer Function 1/3("TF ") -> Format Data  for Workspace/2(Sxy)
  Transfer Function 1/1(TF Mag) -> Sxy Magnitude dB1/1
  "Transfer Function "/3("TF ") -> Format Data  for Workspace/1(Syy)
  sampler2/1 -> Format Data  for Workspace/3(Swap)
  RA/1 -> Switch4/3, Switch5/1  "A"
  Run/1 -> "Transfer Function "/Enable, Transfer Function 1/Enable

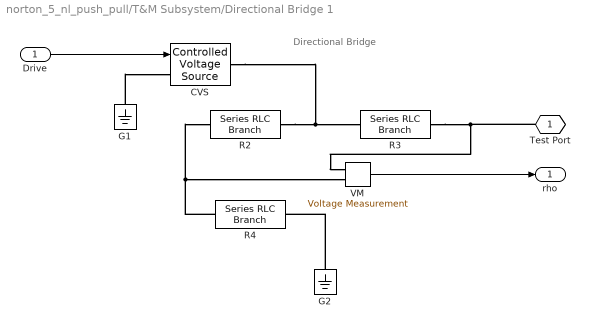
== system norton_5_nl_push_pull/T&M Subsystem/Directional Bridge 1 ==
  note: Directional Bridge
  Drive : Inport  OutDataType=sfix(16)  OutScaling=2^0
  CVS : powerlib/Electrical Sources/Controlled Voltage Source  Description=source block  DialogController=POWERSYS.PowerSysDialog  SystemSampleTime=-1  Initialize=off  Source_Type=AC  Amplitude=0  Phase=0  Frequency=0  Measurements=None
      settings: AttributesFormatString=\n
  G1 : powerlib/Elements/Ground  DialogController=POWERSYS.PowerSysDialog  PhysicalDomain=powersysdomain  SubClassName=unknown  LeftPortType=p1  RightPortType=p1  LConnTagsString=a
  G2 : powerlib/Elements/Ground  DialogController=POWERSYS.PowerSysDialog  PhysicalDomain=powersysdomain  SubClassName=unknown  LeftPortType=p1  RightPortType=p1  LConnTagsString=a
  R2 : powerlib/Elements/Series RLC Branch  DialogController=POWERSYS.PowerSysDialog  PhysicalDomain=powersysdomain  SubClassName=unknown  LeftPortType=p1  RightPortType=p1  LConnTagsString=__new0  RConnTagsString=__new0  BranchType=R  Resistance=Zo  Inductance=1.0  SetiL0=off  InitialCurrent=0  Capacitance=1.0  Setx0=off  InitialVoltage=0  Measurements=None
  R3 : powerlib/Elements/Series RLC Branch  DialogController=POWERSYS.PowerSysDialog  PhysicalDomain=powersysdomain  SubClassName=unknown  LeftPortType=p1  RightPortType=p1  LConnTagsString=__new0  RConnTagsString=__new0  BranchType=R  Resistance=Zo  Inductance=1.0  SetiL0=off  InitialCurrent=0  Capacitance=1.0  Setx0=off  InitialVoltage=0  Measurements=None
  R4 : powerlib/Elements/Series RLC Branch  DialogController=POWERSYS.PowerSysDialog  PhysicalDomain=powersysdomain  SubClassName=unknown  LeftPortType=p1  RightPortType=p1  LConnTagsString=__new0  RConnTagsString=__new0  BranchType=R  Resistance=Zo  Inductance=1.0  SetiL0=off  InitialCurrent=0  Capacitance=1.0  Setx0=off  InitialVoltage=0  Measurements=None
  VM : powerlib/Measurements/Voltage Measurement  Tag=PoWeRsYsTeMmEaSuReMeNt  DialogController=POWERSYS.PowerSysDialog  SystemSampleTime=-1  PhasorSimulation=off  OutputType=Magnitude  PSBequivalent=0
  Test Port : PMIOPort  Tag=PMCPort  Port=1  Side=Right
  rho : Outport  OutDataType=sfix(16)  OutScaling=2^0
  wires:
  VM/1 -> rho/1
  Drive/1 -> CVS/1
  connections:
  R2/RConn1 -- R3/LConn1 -- CVS/RConn1
  R4/LConn1 -- VM/LConn2 -- R2/LConn1
  G2/LConn1 -- R4/RConn1
  R3/RConn1 -- VM/LConn1 -- Test Port/RConn1
  G1/LConn1 -- CVS/LConn1

== system norton_5_nl_push_pull/T&M Subsystem/Directional Bridge 2 ==
  note: Directional Bridge
  Drive : Inport  OutDataType=sfix(16)  OutScaling=2^0
  CVS : powerlib/Electrical Sources/Controlled Voltage Source  Description=source block  DialogController=POWERSYS.PowerSysDialog  SystemSampleTime=-1  Initialize=off  Source_Type=AC  Amplitude=0  Phase=0  Frequency=0  Measurements=None
      settings: AttributesFormatString=\n
  G1 : powerlib/Elements/Ground  DialogController=POWERSYS.PowerSysDialog  PhysicalDomain=powersysdomain  SubClassName=unknown  LeftPortType=p1  RightPortType=p1  LConnTagsString=a
  G2 : powerlib/Elements/Ground  DialogController=POWERSYS.PowerSysDialog  PhysicalDomain=powersysdomain  SubClassName=unknown  LeftPortType=p1  RightPortType=p1  LConnTagsString=a
  R2 : powerlib/Elements/Series RLC Branch  DialogController=POWERSYS.PowerSysDialog  PhysicalDomain=powersysdomain  SubClassName=unknown  LeftPortType=p1  RightPortType=p1  LConnTagsString=__new0  RConnTagsString=__new0  BranchType=R  Resistance=Zo  Inductance=1.0  SetiL0=off  InitialCurrent=0  Capacitance=1.0  Setx0=off  InitialVoltage=0  Measurements=None
  R3 : powerlib/Elements/Series RLC Branch  DialogController=POWERSYS.PowerSysDialog  PhysicalDomain=powersysdomain  SubClassName=unknown  LeftPortType=p1  RightPortType=p1  LConnTagsString=__new0  RConnTagsString=__new0  BranchType=R  Resistance=Zo  Inductance=1.0  SetiL0=off  InitialCurrent=0  Capacitance=1.0  Setx0=off  InitialVoltage=0  Measurements=None
  R4 : powerlib/Elements/Series RLC Branch  DialogController=POWERSYS.PowerSysDialog  PhysicalDomain=powersysdomain  SubClassName=unknown  LeftPortType=p1  RightPortType=p1  LConnTagsString=__new0  RConnTagsString=__new0  BranchType=R  Resistance=Zo  Inductance=1.0  SetiL0=off  InitialCurrent=0  Capacitance=1.0  Setx0=off  InitialVoltage=0  Measurements=None
  VM : powerlib/Measurements/Voltage Measurement  Tag=PoWeRsYsTeMmEaSuReMeNt  DialogController=POWERSYS.PowerSysDialog  SystemSampleTime=-1  PhasorSimulation=off  OutputType=Magnitude  PSBequivalent=0
  Test Port : PMIOPort  Tag=PMCPort  Port=1  Side=Right
  rho : Outport  OutDataType=sfix(16)  OutScaling=2^0
  wires:
  Drive/1 -> CVS/1
  VM/1 -> rho/1
  connections:
  G1/LConn1 -- CVS/LConn1
  Test Port/RConn1 -- VM/LConn1 -- R3/RConn1
  G2/LConn1 -- R4/RConn1
  R2/LConn1 -- VM/LConn2 -- R4/LConn1
  CVS/RConn1 -- R3/LConn1 -- R2/RConn1

== system norton_5_nl_push_pull/T&M Subsystem/Spectrum ==
  Input Signal : Inport  OutDataType=sfix(16)  OutScaling=2^0
  Enable : EnablePort
  Gain : Gain  Gain=1/sqrt(Zo)  ParameterDataType=fixdt(1, 16)  ParameterScaling=2^0  OutDataType=fixdt(1, 16)  OutScaling=2^0
  Spectrum Scope : dspsnks4/Spectrum Scope  DialogController=dspdialog.SpectrumScope  DialogControllerArgs=DataTag13  SystemSampleTime=-1  ScopeProperties=on  Domain=Frequency  HorizSpan=1  UseBuffer=on  BufferSize=512  Overlap=0  inpFftLenInherit=off  FFTlength=128  numAvg=1  DisplayProperties=off  AxisGrid=on  Memory=off  FrameNumber=on  AxisLegend=off  AxisZoom=off  OpenScopeAtSimStart=on  OpenScopeImmediately=off  FigPos=[814 59 408 234]  AxisProperties=off  XUnits=Hertz  XRange=One-sided ([0...Fs/2])  XDisplay=0  InheritXIncr=on  XIncr=1.0  XLabel=Samples  XLimit=Auto  YUnits=dBm  XMax=1  XMin=0  YLabel=dBm  LineProperties=off  wintypeSpecScope=Hann  RsSpecScope=50  betaSpecScope=5  winsampSpecScope=Periodic  XAxisParamsVer=6.9
      settings: YMin=-70  YMax=40
  anti alias : dsparch4/Analog Filter Design  method=Elliptic  filttype=Lowpass  N=8  Wlo=BW*2*pi  Whi=80  Rp=0.11  Rs=100
  sampler : ZeroOrderHold  SampleTime=1/(2.56*BW)
  wires:
  sampler/1 -> Gain/1
  anti alias/1 -> sampler/1
  Input Signal/1 -> anti alias/1
  Gain/1 -> Spectrum Scope/1

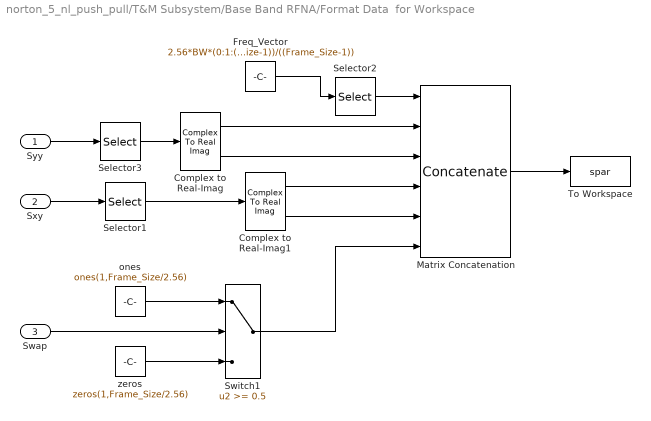
== system norton_5_nl_push_pull/T&M Subsystem/Base Band RFNA/Format Data  for Workspace ==
  Syy : Inport  OutDataType=sfix(16)  OutScaling=2^0
  Sxy : Inport  Port=2  OutDataType=sfix(16)  OutScaling=2^0
  Swap : Inport  Port=3  OutDataType=sfix(16)  OutScaling=2^0
  Complex to Real-Imag : ComplexToRealImag
  Complex to Real-Imag1 : ComplexToRealImag
  Freq_Vector : Constant  Value=2.56*BW*(0:1:(Frame_Size-1))/((Frame_Size-1))  OutDataType=sfix(16)  OutScaling=2^0
  Matrix Concatenation : Concatenate  NumInputs=6  Mode=Multidimensional array  ConcatenateDimension=2
  Selector1 : Selector  InputPortWidth=Frame_Size  IndexOptions=Index vector (dialog)  Indices=[1:Frame_Size/2.56]  OutputSizes=1
  Selector2 : Selector  InputPortWidth=Frame_Size  IndexOptions=Index vector (dialog)  Indices=[1:Frame_Size/2.56]  OutputSizes=1
  Selector3 : Selector  InputPortWidth=Frame_Size  IndexOptions=Index vector (dialog)  Indices=[1:Frame_Size/2.56]  OutputSizes=1
  Switch1 : Switch  Threshold=0.5  SaturateOnIntegerOverflow=on
  To Workspace : ToWorkspace  VariableName=spar  SampleTime=-1  SaveFormat=Array
      settings: MaxDataPoints=1
  ones : Constant  Value=ones(1,Frame_Size/2.56)  OutDataType=sfix(16)  OutScaling=2^0
  zeros : Constant  Value=zeros(1,Frame_Size/2.56)  OutDataType=sfix(16)  OutScaling=2^0
  wires:
  Matrix Concatenation/1 -> To Workspace/1
  Complex to Real-Imag1/2 -> Matrix Concatenation/5
  Freq_Vector/1 -> Selector2/1
  Complex to Real-Imag/1 -> Matrix Concatenation/2
  Complex to Real-Imag/2 -> Matrix Concatenation/3
  Complex to Real-Imag1/1 -> Matrix Concatenation/4
  Syy/1 -> Selector3/1
  Sxy/1 -> Selector1/1
  ones/1 -> Switch1/1
  zeros/1 -> Switch1/3
  Swap/1 -> Switch1/2
  Switch1/1 -> Matrix Concatenation/6
  Selector3/1 -> Complex to Real-Imag/1
  Selector1/1 -> Complex to Real-Imag1/1
  Selector2/1 -> Matrix Concatenation/1

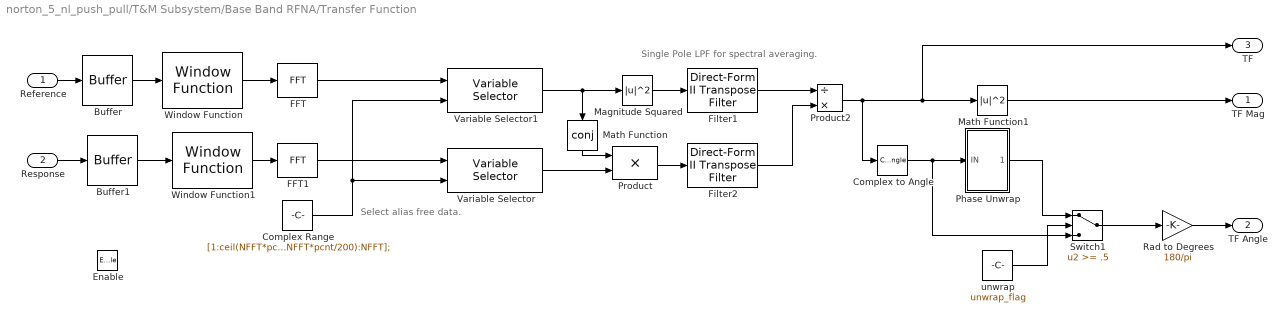
== system norton_5_nl_push_pull/T&M Subsystem/Base Band RFNA/Transfer Function  ==
  note: Select alias free data.
  note: Single Pole LPF for spectral averaging.
  Reference : Inport  OutDataType=sfix(16)  OutScaling=2^0
  Response : Inport  Port=2  OutDataType=sfix(16)  OutScaling=2^0
  Enable : EnablePort
  Buffer : dspbuff3/Buffer  N=NFFT  V=0  ic=0
  Buffer1 : dspbuff3/Buffer  N=NFFT  V=0  ic=0
  Complex Range : Constant  Value=[1:ceil(NFFT*pcnt/200),ceil(1+NFFT-NFFT*pcnt/200):NFFT];  OutDataType=sfix(16)  OutScaling=2^0
  Complex to Angle : ComplexToMagnitudeAngle  Output=Angle
  FFT : dspxfrm3/FFT  DialogController=dspDDGCreate  DialogControllerArgs=DataTag3  CompMethod=Table lookup  TableOpt=NEW  TableOptActive=Speed  BitRevOrder=off  InheritFFTLength=on  FFTLength=64  SkipNorm=on  firstCoeffMode=Specify word length  firstCoeffWordLength=16  firstCoeffFracLength=15  roundingMode=Floor  overflowMode=off
  FFT1 : dspxfrm3/FFT  DialogController=dspDDGCreate  DialogControllerArgs=DataTag4  CompMethod=Table lookup  TableOpt=NEW  TableOptActive=Speed  BitRevOrder=off  InheritFFTLength=on  FFTLength=64  SkipNorm=on  firstCoeffMode=User-defined  firstCoeffWordLength=16  firstCoeffFracLength=15  roundingMode=Floor  overflowMode=off
  Filter1 : dsparch3/Direct-Form II Transpose Filter  num=1  den=[Navg -(Navg-1)]  ic=eps
  Filter2 : dsparch3/Direct-Form II Transpose Filter  num=1  den=[Navg -(Navg-1)]  ic=eps
  Magnitude Squared : Math  Operator=magnitude^2  OutDataType=sfix(16)  OutScaling=2^0  SaturateOnIntegerOverflow=on
  Math Function : Math  Operator=conj  OutDataType=sfix(16)  OutScaling=2^0  SaturateOnIntegerOverflow=on
  Math Function1 : Math  Operator=magnitude^2  OutDataType=sfix(16)  OutScaling=2^0  SaturateOnIntegerOverflow=on
  Phase Unwrap : Subsystem
  Product : Product  OutDataType=sfix(16)  OutScaling=2^0  SaturateOnIntegerOverflow=on  InputSameDT=on  OutDataTypeStr=Inherit: Same as first input
  Product2 : Product  Inputs=/*  OutDataType=sfix(16)  OutScaling=2^0  SaturateOnIntegerOverflow=on  InputSameDT=on  OutDataTypeStr=Inherit: Same as first input
  Rad to Degrees : Gain  Gain=180/pi  ParameterDataType=sfix(16)  ParameterScaling=2^0  OutDataType=sfix(16)  OutScaling=2^0
  Switch1 : Switch  Threshold=.5
  Variable Selector : dspindex/Variable Selector  NumInputs=1  rowsOrCols=Rows  IdxMode=Variable  Elements=[1 3]  ZerOneIdxMode=One-based  errmode=Clip Index  FillMode=on  FillValues=0
  Variable Selector1 : dspindex/Variable Selector  NumInputs=1  rowsOrCols=Rows  IdxMode=Variable  Elements=[1 3]  ZerOneIdxMode=One-based  errmode=Clip Index  FillMode=on  FillValues=0
  Window Function : dspsigops/Window Function  DialogController=dspDDGCreate  DialogControllerArgs=DataTag6  winmode=Apply window to input  wintype=Hann  sampmode=Continuous  samptime=1  N=64  Rs=50  beta=10  winsamp=Periodic  UserWindow=hamming  OptParams=off  UserParams={'symmetric'}  dataType=double  isSigned=on  wordLen=16  udDataType=sfix(16)  fracBitsMode=Best precision  numFracBits=15  roundingMode=Floor  overflowMode=off  numSidelobes=4  sidelobeLevel=-30
  Window Function1 : dspsigops/Window Function  DialogController=dspDDGCreate  DialogControllerArgs=DataTag7  winmode=Apply window to input  wintype=Hann  sampmode=Continuous  samptime=1  N=64  Rs=50  beta=10  winsamp=Periodic  UserWindow=hamming  OptParams=off  UserParams={'symmetric'}  dataType=double  isSigned=on  wordLen=16  udDataType=sfix(16)  fracBitsMode=Best precision  numFracBits=15  roundingMode=Floor  overflowMode=off  numSidelobes=4  sidelobeLevel=-30
  unwrap : Constant  Value=unwrap_flag  OutDataType=sfix(16)  OutScaling=2^0
  TF Mag : Outport  OutDataType=sfix(16)  OutScaling=2^0
  TF Angle : Outport  Port=2  OutDataType=sfix(16)  OutScaling=2^0
  "TF " : Outport  Port=3  OutDataType=sfix(16)  OutScaling=2^0
  wires:
  Phase Unwrap/1(Out1) -> Switch1/1
  unwrap/1 -> Switch1/2
  Switch1/1 -> Rad to Degrees/1
  Variable Selector1/1 -> Math Function/1, Magnitude Squared/1
  Variable Selector/1 -> Product/2
  Product2/1 -> Complex to Angle/1, Math Function1/1, "TF "/1
  Buffer1/1 -> Window Function1/1
  Buffer/1 -> Window Function/1
  Filter2/1 -> Product2/2
  Filter1/1 -> Product2/1
  Window Function1/1 -> FFT1/1
  Window Function/1 -> FFT/1
  Math Function1/1 -> TF Mag/1
  FFT/1 -> Variable Selector1/1
  Magnitude Squared/1 -> Filter1/1
  Math Function/1 -> Product/1
  FFT1/1 -> Variable Selector/1
  Product/1 -> Filter2/1
  Reference/1 -> Buffer/1
  Response/1 -> Buffer1/1
  Rad to Degrees/1 -> TF Angle/1
  Complex to Angle/1 -> Phase Unwrap/1(IN), Switch1/3
  Complex Range/1 -> Variable Selector1/2, Variable Selector/2
